simulink model "getPWM"  (R2012b)
settings: Solver=FixedStepDiscrete  StartTime=0.0  StopTime=inf  FixedStep=0.01  RelTol=1e-3
libraries: WBCLibrary x3
settings Model: Creator=daniele  LastModifiedBy=daniele

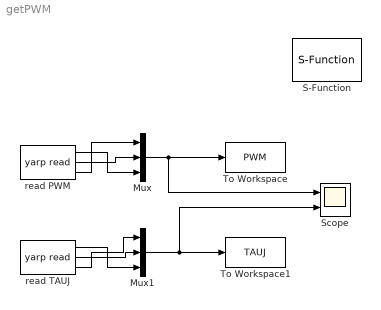
== system getPWM ==
  Mux : Mux  Inputs=3
  Mux1 : Mux  Inputs=3
  S-Function : WBCLibrary/Utilities/S-Function  rate=0.010
  Scope : Scope  NumInputPorts=2
      settings: TimeRange=25  YMin=-250~-15  YMax=325~15
  To Workspace : ToWorkspace  VariableName=PWM  SampleTime=-1  SaveFormat=Timeseries
  To Workspace1 : ToWorkspace  VariableName=TAUJ  SampleTime=-1  SaveFormat=Timeseries
  read PWM : WBCLibrary/Utilities/yarp read  from=['/controlBoardDumper/torso/getOutputs']  to='...'  num=3
  read TAUJ : WBCLibrary/Utilities/yarp read  from=['/wholeBodyDynamicsTree/torso/Torques:o']  to='...'  num=3
  wires:
  read PWM/2 -> Mux/2
  read PWM/1 -> Mux/3
  read PWM/3 -> Mux/1
  read TAUJ/1 -> Mux1/3
  read TAUJ/3 -> Mux1/1
  read TAUJ/2 -> Mux1/2
  Mux/1 -> Scope/1, To Workspace/1
  Mux1/1 -> Scope/2, To Workspace1/1
